simulink model "LC_dynamic_tau_test"  (R2023a)
settings: Solver=VariableStepAuto  StartTime=0.0  StopTime=10.0  RelTol=1e-3
settings Model: Creator=28303  LastModifiedBy=28303

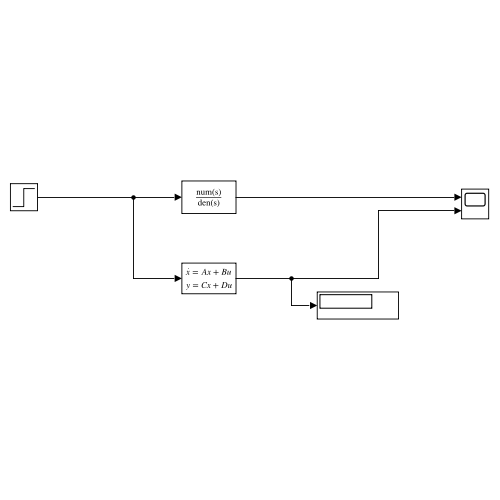
[thumbnail: Simulink's stored preview of the top-level diagram]
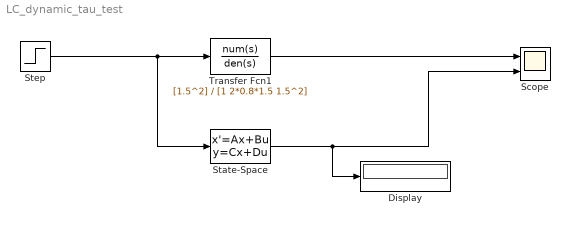
== system LC_dynamic_tau_test ==
  Display : Display
  Scope : Scope  NumInputPorts=2
  State-Space : StateSpace  A=[0 -2.25;1 -2.4]  B=[2.25;0]  C=eye(2)  D=[0;0]  InitialCondition=[0 0]
  Step : Step  SampleTime=0
  Transfer Fcn1 : TransferFcn  Numerator=[1.5^2]  Denominator=[1 2*0.8*1.5 1.5^2]
  wires:
  Step/1 -> State-Space/1, Transfer Fcn1/1
  Transfer Fcn1/1 -> Scope/1
  State-Space/1 -> Display/1, Scope/2
